simulink model "Analytical_freq_sim"  (Simulink 6.3)
settings: Solver=ode23s  StartTime=0  StopTime=400  MaxStep=0.1  RelTol=1e-3
undefined symbols (not defined in the file or in its folder): sigbuilder_block
Description:
  | This is a model of depression in synapses
settings Model: Creator=chchlee  LastModifiedBy=Owner  ExtModeAutoUpdateStatusClock=off  StrictBusMsg=None
settings DataIOCC: SignalLoggingName=sigsOut
settings OptimizationCC: InlineInvariantSignals=on
settings DebuggingCC: SolverPrmCheckMsg=none
settings HardwareCC: TargetUnknown=on
settings GRTTargetCC: ModelReferenceCompliant=off  MatFileLogging=off

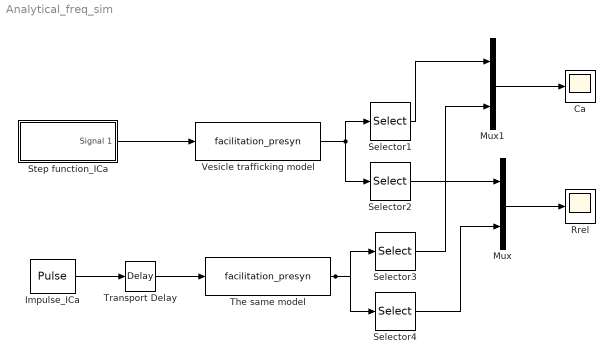
== system Analytical_freq_sim ==
  Ca : Scope
      settings: YMin=-67.5  YMax=-63  SaveName=SteadyState_Cass  DataFormat=Array
  Impulse_ICa : DiscretePulseGenerator  PulseType=Time based  Period=1000/50  PulseWidth=0.1*50
  Mux : Mux  Inputs=2
  Mux1 : Mux  Inputs=2
  Rrel : Scope
      settings: YMin=0.2  YMax=0.95  SaveName=SteadyState_Rrelss  DataFormat=Array
  Selector1 : Selector  Elements=[1]  InputPortWidth=4
  Selector2 : Selector  Elements=[2]  InputPortWidth=4
  Selector3 : Selector  Elements=[1]  InputPortWidth=4
  Selector4 : Selector  Elements=[2]  InputPortWidth=4
  Step function_ICa : Subsystem  Tag=STV Subsys  LoadFcn=sigbuilder_block('load');  StartFcn=sigbuilder_block('start');  StopFcn=sigbuilder_block('stop');  ClipboardFcn=sigbuilder_block('clipboard');  mask(Sigbuilder block){}
      mask help: Sigbuilder GUI
      mask init:
      | if ~strcmp(get_param(bdroot(gcbh),'SimulationStatus'),'stopped') tuvar = sigbuilder_block('maskInit'); end
      settings: CopyFcn=sigbuilder_block('copy');  DeleteFcn=sigbuilder_block('delete');  ModelCloseFcn=sigbuilder_block('modelClose');  PreSaveFcn=sigbuilder_block('preSave');  NameChangeFcn=sigbuilder_block('namechange');  OpenFcn=sigbuilder_block('open',[163.5 66.75 550.5 252.75 ]);  CloseFcn=sigbuilder_block('close');
      mask Display: plot(0,0,100,100,[10,10,40,40,10],[80,20,20,80,80],[40,10],[50,50], [40,27,10],[65,72,56],[40,25,25,10],[28,28,43,43]);
  The same model : S-Function  FunctionName=facilitation_presyn
  Transport Delay : TransportDelay  DelayTime=40  BufferSize=2000
  Vesicle trafficking model : S-Function  FunctionName=facilitation_presyn
  wires:
  Selector2/1 -> Mux/1
  Selector1/1 -> Mux1/1
  Vesicle trafficking model/1 -> Selector1/1, Selector2/1
  Step function_ICa/1(Signal 1) -> Vesicle trafficking model/1
  Transport Delay/1 -> The same model/1
  Mux1/1 -> Ca/1
  Mux/1 -> Rrel/1
  The same model/1 -> Selector3/1, Selector4/1
  Selector3/1 -> Mux1/2
  Selector4/1 -> Mux/2
  Impulse_ICa/1 -> Transport Delay/1

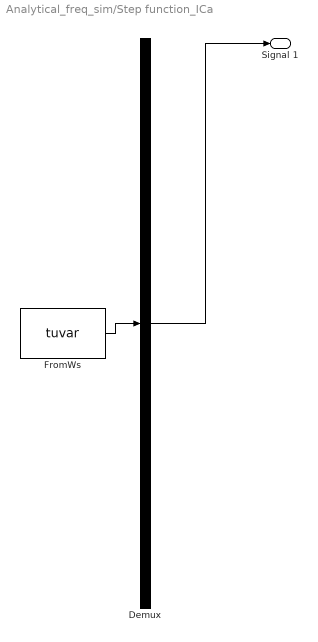
== system Analytical_freq_sim/Step function_ICa ==
  Demux : Demux  Tag=STV Demux  Outputs=1
  FromWs : FromWorkspace  Tag=STV FromWs  VariableName=tuvar  SampleTime=0  SigBuilderData=DataTag0  VnvData=DataTag1
      SigBuilderData=|
      | channels.label = 'Signal 1'
      | channels.allXData = {[0 40 40 100]}
      | channels.allYData = {[0 0 0.05 0.05]}
      | common.afterFinalStr = 'Extrapolate'
      | common.sampleTime = 0
      | dataSet.timeRange = [0 100]
      | dataSet.name = 'Group 1'
  Signal 1 : Outport  Tag=STV Outport
  wires:
  Demux/1 -> Signal 1/1
  FromWs/1 -> Demux/1
